simulink model "cartControl"  (R2014a)
settings: Solver=ode45  StartTime=0.0  StopTime=10.0  RelTol=1e-3
StopFcn:
  | if(exist('Q'))
  | 
  | pause_time = 0.001;
  | pause_on = 1;
  | 
  | figure(2)
  | h=uicontrol(gcf,'style','pushbutton','String','PLAY','position',[175 5 200 30]);
  | set(h,'callback','if(pause_on == 1); for i=1:size(Q.Data,1); plot(Rob, Q.Data(i,:));pause(pause_time); end; end; if(pause_on == 0); for i=1:size(Q.Data,1) plot(Rob, Q.Data(i,:)); end; end;');
  | 
  | h=uicontrol(gcf,'style','pushbutton','String','make slower','position',[50 5 100 30]);
  | set(h,'callback','pause_time = pause_time*2; if(pause_time>1e-4) pause_on = 1; end');
  | 
  | h=uicontrol(gcf,'style','pushbutton','String','make faster','position',[400 5 100 30]);
  | set(h,'callback','if(pause_time<1e-4) pause_on = 0; else; pause_time = pause_time/2; end ');
  | 
  | set(gcf, 'toolbar', 'figure')
  | 
  | end
undefined symbols (not defined in the file or in its folder): fkine, jacob0, transl
undefined symbols (not defined in the file): Rob
settings Model: Creator=user  LastModifiedBy=Wolfgang
settings DebuggingCC: UnderspecifiedInitializationDetection=Classic

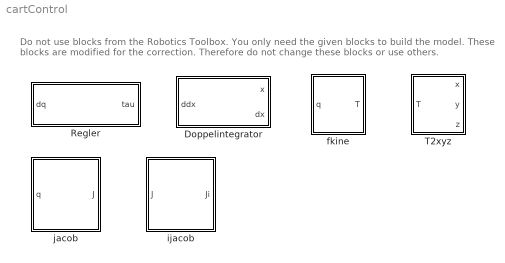
== system cartControl ==
  note: Do not use blocks from the Robotics Toolbox. You only need the given blocks to build the model.
      | These blocks are modified for the correction. Therefore do not change these blocks or use others.
  Doppelintegrator : Subsystem  LoadFcn=set_param(gcb,'Name','Doppelintegrator');  InitFcn=set_param(gcb,'Name','Doppelintegrator');
      mask Display: dpoly([1],[1 0 0], 's')
  Regler : Subsystem  LoadFcn=set_param(gcb,'Name','Regler');  InitFcn=set_param(gcb,'Name','Regler');
      mask Display: disp('PD-Regler')
  T2xyz : Subsystem  LoadFcn=set_param(gcb,'Name','T2xyz');  InitFcn=set_param(gcb,'Name','T2xyz');
      mask help: Convert transform to xyz scalars
  fkine : Subsystem  LoadFcn=set_param(gcb,'Name','fkine');  InitFcn=|  mask{robot=Rob}
      | set_param(gcb,'Name','fkine');
      | 
      | if(~any(strcmp(who,'Testumgebung')))
      | 
      | if(~strcmp(get_param(gcb,'Robot'),'Rob'))
      | set_param(gcb,'Robot','Rob');
      | warning('Verändern sie nichts in der Funktion fkine.')
      | end
      | 
      | end
      mask prompts: robot "SerialLink object"
      mask help: Robot forward kinematics.
      mask Help: Compute homogeneous transform for robot end-effector given joint angles.
      mask Display:
      | port_label('input', 1, 'q')
      | port_label('output', 1, 'T')
      | text(0.9, 0.9, robot.name,  'horizontalAlignment', 'right')
  ijacob : Subsystem  LoadFcn=set_param(gcb,'Name','ijacob');  InitFcn=set_param(gcb,'Name','ijacob');
      mask help: Robot pseudoinverse Jacobian for world coordinates.
      mask Display:
      | text(0.4, 0.7, 'J', 'verticalAlignment', 'top', 'horizontalAlignment', 'left')
      | text(0.65, 0.65, '-1', 'verticalAlignment', 'bottom', 'horizontalAlignment', 'right')
      | port_label('input', 1, 'J');
      | port_label('output', 1, 'Ji')
  jacob : Subsystem  LoadFcn=set_param(gcb,'Name','jacob');  InitFcn=|  mask{robot=Rob}
      | set_param(gcb,'Name','jacob');
      | 
      | if(~any(strcmp(who,'Testumgebung')))
      | 
      | if(~strcmp(get_param(gcb,'Robot'),'Rob'))
      | set_param(gcb,'Robot','Rob');
      | warning('Verändern sie nichts in der Funktion jacob.')
      | end
      | 
      | end
      mask prompts: robot "SerialLink object"
      mask help: Robot Jacobian for end-effector coordinates
      mask init:
      | n=robot.n;
      mask Display:
      | text(0.4, 0.7, 'J', 'verticalAlignment', 'top', 'horizontalAlignment', 'left')
      | text(0.4, 0.7, '0', 'verticalAlignment', 'bottom', 'horizontalAlignment', 'right')
      | text(0.5, 0.2, robot.name,  'horizontalAlignment', 'center')
      | port_label('input', 1, 'q')
      | port_label('output', 1, 'J')

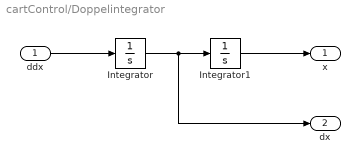
== system cartControl/Doppelintegrator ==
  ddx : Inport
  Integrator : Integrator  InitialCondition=[0 0 0]'
  Integrator1 : Integrator  InitialCondition=[-26.3845 62.7207 -36.3362]'/180*pi
  x : Outport
  dx : Outport  Port=2
  wires:
  Integrator/1 -> dx/1, Integrator1/1
  Integrator1/1 -> x/1
  ddx/1 -> Integrator/1

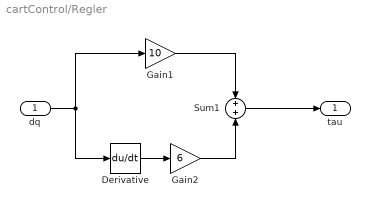
== system cartControl/Regler ==
  dq : Inport
  Derivative : Derivative
  Gain1 : Gain  Gain=10
  Gain2 : Gain  Gain=6
  Sum1 : Sum  Inputs=+|+
  tau : Outport
  wires:
  Sum1/1 -> tau/1
  Gain1/1 -> Sum1/1
  Gain2/1 -> Sum1/2
  dq/1 -> Derivative/1, Gain1/1
  Derivative/1 -> Gain2/1

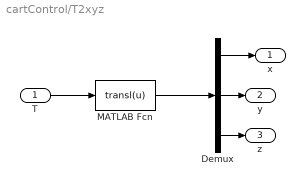
== system cartControl/T2xyz ==
  T : Inport
  Demux : Demux  Outputs=3
  MATLAB Fcn : MATLABFcn  MATLABFcn=transl(u)  OutputDimensions=3
  x : Outport
  y : Outport  Port=2
  z : Outport  Port=3
  wires:
  Demux/3 -> z/1
  Demux/2 -> y/1
  Demux/1 -> x/1
  MATLAB Fcn/1 -> Demux/1
  T/1 -> MATLAB Fcn/1

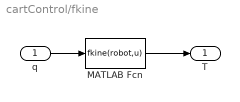
== system cartControl/fkine ==
  q : Inport
  MATLAB Fcn : MATLABFcn  MATLABFcn=fkine(robot,u)  OutputDimensions=[4 4]  Output1D=off
  T : Outport
  wires:
  MATLAB Fcn/1 -> T/1
  q/1 -> MATLAB Fcn/1

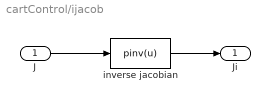
== system cartControl/ijacob ==
  J : Inport
  inverse jacobian : MATLABFcn  MATLABFcn=pinv(u)  Output1D=off
  Ji : Outport
  wires:
  J/1 -> inverse jacobian/1
  inverse jacobian/1 -> Ji/1

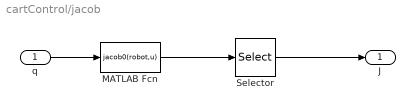
== system cartControl/jacob ==
  q : Inport
  MATLAB Fcn : MATLABFcn  MATLABFcn=jacob0(robot,u)  OutputDimensions=[6 n]  Output1D=off
  Selector : Selector  NumberOfDimensions=2  InputPortWidth=3  IndexOptions=Index vector (dialog),Index vector (dialog)  Indices=[1 2 6],[1 2 3]  OutputSizes=1,1
  J : Outport
  wires:
  q/1 -> MATLAB Fcn/1
  MATLAB Fcn/1 -> Selector/1
  Selector/1 -> J/1
